simulink model "reactor_test_ideal_gas_models_comparison_sim"  (R2017b)
settings: Solver=ode23tb  StartTime=0.0  StopTime=1400  MaxStep=0.2  RelTol=1e-3
libraries: thermochemical x5, simulink x1
settings Model: Creator=ferru  LastModifiedBy=fferrucc
settings SolverCC: AlgebraicLoopSolver=LineSearch

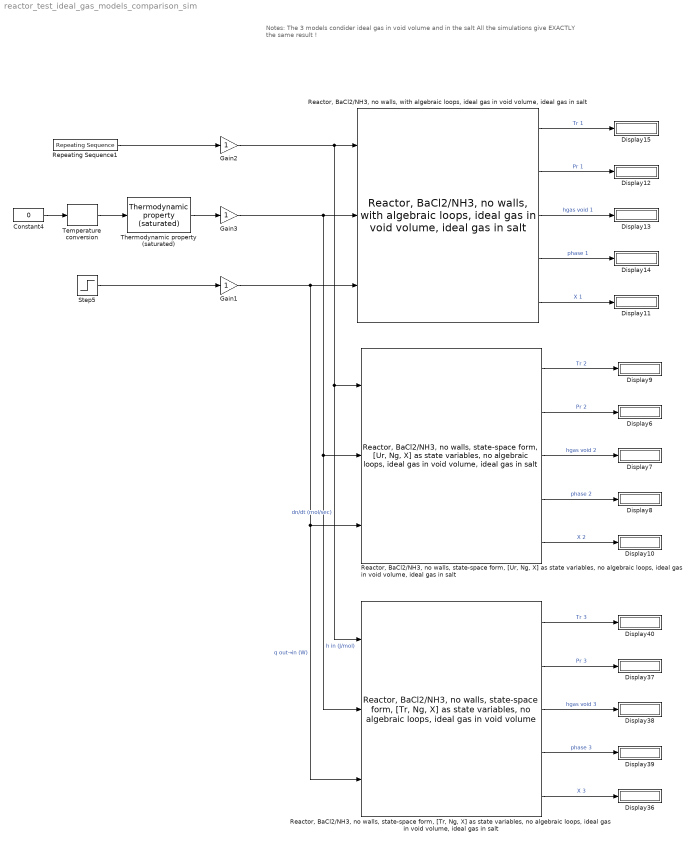
== system reactor_test_ideal_gas_models_comparison_sim ==
  note: Notes:
      | The 3 models condider ideal gas in void volume and in the salt
      | All the simulations give EXACTLY the same result !
  Constant4 : Constant  Value=0
  Display{6..15,36..40} (15 alike) : Display
  Gain1 : Gain
  Gain2 : Gain
  Gain3 : Gain
  "Reactor, BaCl2/NH3, no walls, state-space form, [Tr, Ng, X] as state variables, no algebraic loops, ideal gas in void volume, ideal gas in salt" : thermochemical/Reactors/Reactor, BaCl2//NH3, state-space form, [Tr, Ng, X] as state variables, no algebraic loops, ideal gas in void volume, ideal gas in salt/Reactor, BaCl2//NH3, no walls, state-space form, [Tr, Ng, X] as state variables, no algebraic loops,  ideal gas in void volume  pairName=Barium chloride/Ammonia (BaCl2/NH3)  gasName=Ammonia gas (NH3)  binderName=ENG  N_salt=N_salt  N_binder=N_binder  K_cin=K_cin  V_void=V_void  fluid=fluid  Tr_init=Tr_init  X_init=X_init  N_gas_free_volume_init=N_gas_free_volume_init  m_composite_kg=3.223  m_salt_kg=2.385  m_binder_kg=0.83797  m_gas_when_reactor_fully_charged=1.5605  T_ref=239.8236  u_gas_at_T_ref=-1994.0066  U_binder_at_T_ref=0  U_salt_at_X0_T_ref=0  R=8.3145  cP_gas=42.5775  cV_gas=29.4370  nu=8  cP_s0=75.1  dh_r_0=38250  M_binder=0.012011  cP_binder=714.36  P_dead_zone=0.0001  dn_dead_zone=0.0001
      settings: SourceProductName=@ Thermochemical
  "Reactor, BaCl2/NH3, no walls, state-space form, [Ur, Ng, X] as state variables, no algebraic loops, ideal gas in void volume, ideal gas in salt" : thermochemical/Reactors/Reactor, BaCl2//NH3, state-space form, [Ur, Ng, X] as state variables, no algebraic loops, ideal gas in void volume, ideal gas in salt/Reactor, BaCl2//NH3, no walls, state-space form, [Ur, Ng, X] as state variables, no algebraic loops, ideal gas in void volume, ideal gas in salt  pairName=Barium chloride/Ammonia (BaCl2/NH3)  gasName=Ammonia gas (NH3)  binderName=ENG  N_salt=N_salt  N_binder=N_binder  K_cin=K_cin  V_void=V_void  Tr_init=Tr_init  X_init=X_init  N_gas_free_volume_init=N_gas_free_volume_init  m_composite_kg=3.223  m_salt_kg=2.385  m_binder_kg=0.83797  m_gas_when_reactor_fully_charged=1.5605  T_ref=239.8236  u_gas_at_T_ref=-1994.0066  U_binder_at_T_ref=0  U_salt_at_X0_T_ref=0  R=8.3145  cP_gas=42.5775  nu=8  cP_s0=75.1  dh_r_0=38250  M_binder=0.012011  cP_binder=714.36  P_dead_zone=0.0001  dn_dead_zone=0.0001
      settings: SourceProductName=@ Thermochemical
  "Reactor, BaCl2/NH3, no walls, with algebraic loops, ideal gas in void volume, ideal gas in salt" : thermochemical/Reactors/Reactor, BaCl2//NH3, with algebraic loops, ideal gas in void volume, ideal gas in salt/Reactor, BaCl2//NH3, no walls, with algebraic loops, ideal gas in void volume, ideal gas in salt  pairName=Barium chloride/Ammonia (BaCl2/NH3)  gasName=Ammonia gas (NH3)  binderName=ENG  N_salt=N_salt  N_binder=N_binder  K_cin=K_cin  V_void=V_void  fluid=fluid  Tr_init=Tr_init  X_init=X_init  N_gas_free_volume_init=N_gas_free_volume_init  m_composite_kg=3.223  m_salt_kg=2.385  m_binder_kg=0.83797  m_gas_when_reactor_fully_charged=1.5605  T_ref=239.8236  u_gas_at_T_ref=-1994.0066  U_binder_at_T_ref=0  U_salt_at_X0_T_ref=0  cP_gas=42.5775  nu=8  cP_s0=75.1  Pr_0=1e-05  dh_r_0=38250  ds_r_0=232.38  M_binder=0.012011  cP_binder=714.36  P_dead_zone=0.0001  dn_dead_zone=0.0001  R=8.3145
      settings: SourceProductName=@ Thermochemical
  Repeating Sequence1 : simulink/Sources/Repeating Sequence  rep_seq_t=[0, 1, 1.001, 1.1, 1.1001, 1.2, 1.2002, 1.3, 1.3001]*1e3  rep_seq_y=[0, 0, 1, 1, 0, 0, 1, 1, 0]*(-0.01)
  Step5 : Step  Time=1200  After=+1000  SampleTime=0
  Temperature conversion : thermochemical/Conversions/Temperature conversion  sel=°C --> K
      settings: SourceProductName=@ Thermochemical
  Thermodynamic property (saturated) : thermochemical/Thermodynamic fluid properties/Thermodynamic  property (saturated)  sel=h(T) vap. (J/mol)  fluid=fluid  lookup1D_BreakPoint1=fluid.sat.T  lookup1D_Data=fluid.sat.vap.h_molar
      settings: SourceProductName=@ Thermochemical
  wires:
  "Reactor, BaCl2/NH3, no walls, state-space form, [Ur, Ng, X] as state variables, no algebraic loops, ideal gas in void volume, ideal gas in salt"/5 -> Display10/1  "X 2"
  "Reactor, BaCl2/NH3, no walls, state-space form, [Ur, Ng, X] as state variables, no algebraic loops, ideal gas in void volume, ideal gas in salt"/4 -> Display8/1  "phase 2"
  "Reactor, BaCl2/NH3, no walls, state-space form, [Ur, Ng, X] as state variables, no algebraic loops, ideal gas in void volume, ideal gas in salt"/3 -> Display7/1  "hgas void 2"
  "Reactor, BaCl2/NH3, no walls, state-space form, [Ur, Ng, X] as state variables, no algebraic loops, ideal gas in void volume, ideal gas in salt"/2 -> Display6/1  "Pr 2"
  "Reactor, BaCl2/NH3, no walls, state-space form, [Ur, Ng, X] as state variables, no algebraic loops, ideal gas in void volume, ideal gas in salt"/1 -> Display9/1  "Tr 2"
  "Reactor, BaCl2/NH3, no walls, with algebraic loops, ideal gas in void volume, ideal gas in salt"/1 -> Display15/1  "Tr 1"
  "Reactor, BaCl2/NH3, no walls, with algebraic loops, ideal gas in void volume, ideal gas in salt"/2 -> Display12/1  "Pr 1"
  "Reactor, BaCl2/NH3, no walls, with algebraic loops, ideal gas in void volume, ideal gas in salt"/3 -> Display13/1  "hgas void 1"
  "Reactor, BaCl2/NH3, no walls, with algebraic loops, ideal gas in void volume, ideal gas in salt"/4 -> Display14/1  "phase 1"
  "Reactor, BaCl2/NH3, no walls, with algebraic loops, ideal gas in void volume, ideal gas in salt"/5 -> Display11/1  "X 1"
  Temperature conversion/1 -> Thermodynamic property (saturated)/1
  Constant4/1 -> Temperature conversion/1
  Gain2/1 -> "Reactor, BaCl2/NH3, no walls, state-space form, [Tr, Ng, X] as state variables, no algebraic loops, ideal gas in void volume, ideal gas in salt"/1, "Reactor, BaCl2/NH3, no walls, state-space form, [Ur, Ng, X] as state variables, no algebraic loops, ideal gas in void volume, ideal gas in salt"/1, "Reactor, BaCl2/NH3, no walls, with algebraic loops, ideal gas in void volume, ideal gas in salt"/1  "dn/dt (mol/sec)"
  Gain1/1 -> "Reactor, BaCl2/NH3, no walls, state-space form, [Tr, Ng, X] as state variables, no algebraic loops, ideal gas in void volume, ideal gas in salt"/3, "Reactor, BaCl2/NH3, no walls, state-space form, [Ur, Ng, X] as state variables, no algebraic loops, ideal gas in void volume, ideal gas in salt"/3, "Reactor, BaCl2/NH3, no walls, with algebraic loops, ideal gas in void volume, ideal gas in salt"/3  "q out→in (W)"
  Gain3/1 -> "Reactor, BaCl2/NH3, no walls, state-space form, [Tr, Ng, X] as state variables, no algebraic loops, ideal gas in void volume, ideal gas in salt"/2, "Reactor, BaCl2/NH3, no walls, state-space form, [Ur, Ng, X] as state variables, no algebraic loops, ideal gas in void volume, ideal gas in salt"/2, "Reactor, BaCl2/NH3, no walls, with algebraic loops, ideal gas in void volume, ideal gas in salt"/2  "h in (J/mol)"
  "Reactor, BaCl2/NH3, no walls, state-space form, [Tr, Ng, X] as state variables, no algebraic loops, ideal gas in void volume, ideal gas in salt"/3 -> Display38/1  "hgas void 3"
  "Reactor, BaCl2/NH3, no walls, state-space form, [Tr, Ng, X] as state variables, no algebraic loops, ideal gas in void volume, ideal gas in salt"/2 -> Display37/1  "Pr 3"
  "Reactor, BaCl2/NH3, no walls, state-space form, [Tr, Ng, X] as state variables, no algebraic loops, ideal gas in void volume, ideal gas in salt"/4 -> Display39/1  "phase 3"
  "Reactor, BaCl2/NH3, no walls, state-space form, [Tr, Ng, X] as state variables, no algebraic loops, ideal gas in void volume, ideal gas in salt"/5 -> Display36/1  "X 3"
  "Reactor, BaCl2/NH3, no walls, state-space form, [Tr, Ng, X] as state variables, no algebraic loops, ideal gas in void volume, ideal gas in salt"/1 -> Display40/1  "Tr 3"
  Thermodynamic property (saturated)/1 -> Gain3/1
  Step5/1 -> Gain1/1
  Repeating Sequence1/1 -> Gain2/1
